simulink model "block"  (R2025a)
settings: Solver=ode45  StartTime=0  StopTime=3  MaxStep=0.001  RelTol=1e-3
settings Model: Creator=Alex_  LastModifiedBy=Alex_
settings DataIOCC: LimitDataPoints=on  MaxDataPoints=3000

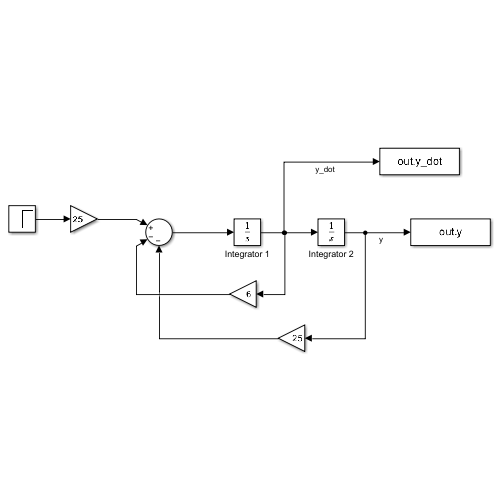
[thumbnail: Simulink's stored preview of the top-level diagram]
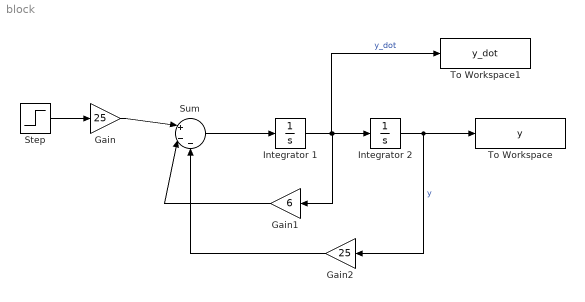
== system block ==
  Gain : Gain  Gain=25
  Gain1 : Gain  Gain=6
  Gain2 : Gain  Gain=25
  Integrator 1 : Integrator
  Integrator 2 : Integrator
  Step : Step  Time=0  SampleTime=0
  Sum : Sum  Inputs=|+--
  To Workspace : ToWorkspace  VariableName=y  SampleTime=-1
      settings: MaxDataPoints=3000
  To Workspace1 : ToWorkspace  VariableName=y_dot  SampleTime=-1
      settings: MaxDataPoints=3000
  wires:
  Step/1 -> Gain/1
  Gain/1 -> Sum/1
  Sum/1 -> Integrator 1/1
  Integrator 1/1 -> To Workspace1/1, Gain1/1, Integrator 2/1  "y_dot"
  Integrator 2/1 -> Gain2/1, To Workspace/1  "y"
  Gain2/1 -> Sum/3
  Gain1/1 -> Sum/2
